simulink model "ROS_example"  (R2026a)
settings: Solver=FixedStepDiscrete  StopTime=tspan  FixedStep=dt_sim
values from neighbouring files (symbols this model uses):
  A = [0 1;-k/m -b/m]    [init_ROS_example.m]
  B = [0;1]    [init_ROS_example.m]
  dt_control = roundToSimTimestep(0.01,dt_sim)    [init_ROS_example.m]
  dt_data = roundToSimTimestep(1/30,dt_sim)    [init_ROS_example.m]
  dt_sim = 0.001    [init_ROS_example.m]
  x0 = [0;0]    [init_ROS_example.m]
  x_u = 1    [init_ROS_example.m]
undefined symbols (not defined in the file or in its folder): DiscIntNeverNeededParam, PID
libraries: ros2lib x6, slpidlib x1
settings Model: Creator=koryh  LastModifiedBy=koryh

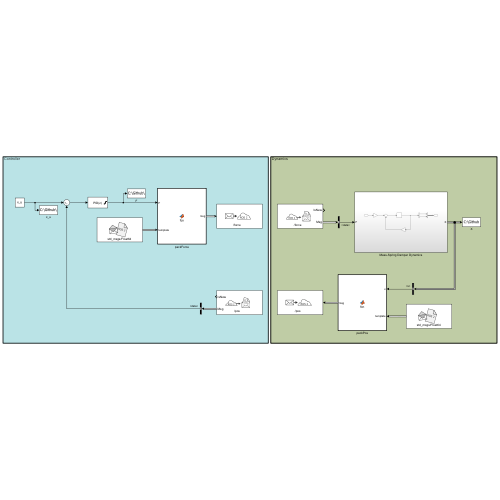
[thumbnail: Simulink's stored preview of the top-level diagram]
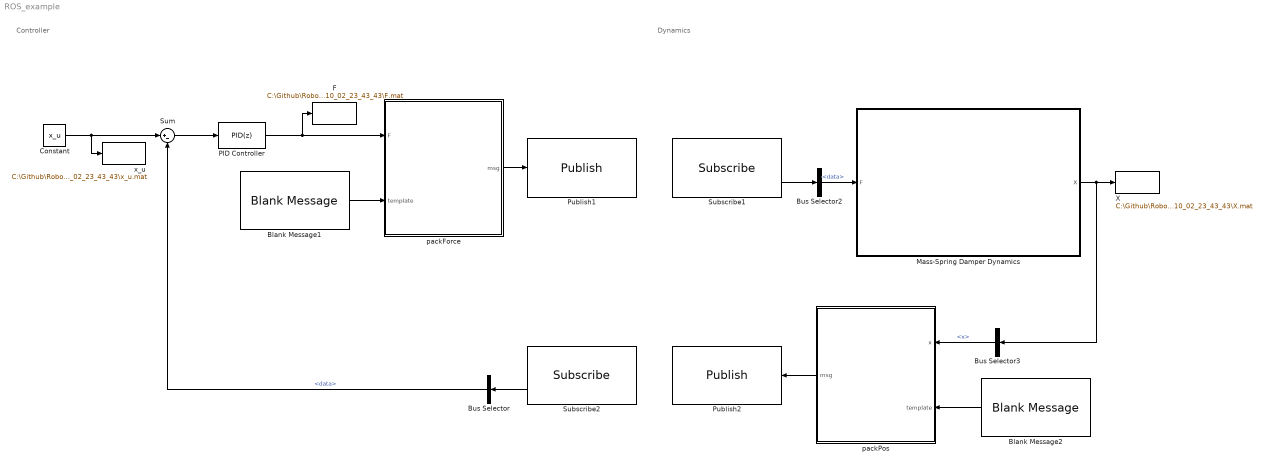
== system ROS_example ==
  note: Controller
  note: Dynamics
  Blank Message1 : ros2lib/Blank Message  messageClass=Message  entityType=std_msgs/Float64  messageType=std_msgs/Float64  SampleTime=0.01
  Blank Message2 : ros2lib/Blank Message  messageClass=Message  entityType=std_msgs/Float64  messageType=std_msgs/Float64  SampleTime=0.01
  Bus Selector : BusSelector  OutputSignals=data
  Bus Selector2 : BusSelector  OutputSignals=data
  Bus Selector3 : BusSelector  OutputSignals=x
  Constant : Constant  Value=x_u
  F : ToFile  Filename=C:\Github\Robosub\controls-onboarding-2027\examples\ROS Example\ROS_example_data\2026_10_02_23_43_43\F.mat  MatrixName=F  SaveFormat=Timeseries  SampleTime=dt_data
  Mass-Spring Damper Dynamics : Subsystem
  PID Controller : slpidlib/PID Controller  Controller=PID  Form=Parallel  TimeDomain=Discrete-time  UseExternalTs=off  SampleTime=dt_control  IntegratorMethod=Forward Euler  FilterMethod=Forward Euler  ControllerParametersSource=internal  P=PID.P  I=PID.I  UseKiTs=off  D=PID.D  UseExternalDerivativeSource=off  N=PID.N  UseFilter=on  TunerSelectOption=Transfer Function Based (PID Tuner App)  InitialConditionSource=internal  InitialConditionForIntegrator=0  InitialConditionForFilter=0  DifferentiatorICPrevScaledInput=0  ExternalReset=none  TrackingMode=off  Kt=1  LimitOutput=on  SatLimitsSource=internal  UpperSaturationLimit=PID.output_sat  LowerSaturationLimit=-PID.output_sat  LinearizeAsGain=on  AntiWindupMode=none  Kb=1  LimitIntegrator=off  UpperIntegratorSaturationLimit=inf  LowerIntegratorSaturationLimit=-inf  POutMin=[]  POutMax=[]  IOutMin=[]  IOutMax=[]  DOutMin=[]  DOutMax=[]  NOutMin=[]  NOutMax=[]  SumOutMin=[]  SumOutMax=[]  SaturationOutMin=[]  SaturationOutMax=[]  PParamMin=[]  PParamMax=[]  IParamMin=[]  IParamMax=[]  DParamMin=[]  DParamMax=[]  NParamMin=[]  NParamMax=[]  KbParamMin=[]  KbParamMax=[]  KtParamMin=[]  KtParamMax=[]  KbOutMin=[]  KbOutMax=[]  KtOutMin=[]  KtOutMax=[]  IntegratorOutMin=[]  IntegratorOutMax=[]  FilterOutMin=[]  FilterOutMax=[]  SumI1OutMin=[]  SumI1OutMax=[]  SumI2OutMin=[]  SumI2OutMax=[]  SumI3OutMin=[]  SumI3OutMax=[]  SumI4OutMin=[]  SumI4OutMax=[]  SumDOutMin=[]  SumDOutMax=[]  DifferentiatorOutMin=[]  DifferentiatorOutMax=[]  FilterDiffOutCoefMin=[]  FilterDiffOutCoefMax=[]  ReciprocalOutMin=[]  ReciprocalOutMax=[]  SumDenOutMin=[]  SumDenOutMax=[]  SumNumOutMin=[]  SumNumOutMax=[]  DivideOutMin=[]  DivideOutMax=[]  UdiffTsProdOutMin=[]  UdiffTsProdOutMax=[]  NTsProdOutMin=[]  NTsProdOutMax=[]  UintegralTsProdOutMin=[]  UintegralTsProdOutMax=[]  UngainTsProdOutMin=[]  UngainTsProdOutMax=[]  ClampingZeroOutDataTypeStr=Inherit: Inherit via back propagation  ClampingZeroOutMin=[]  ClampingZeroOutMax=[]  FilterDenConstantOutDataTypeStr=Inherit: Inherit via back propagation  FilterDenConstantOutMin=[]  FilterDenConstantOutMax=[]  PCopyOutDataTypeStr=Inherit: Inherit via back propagation  PCopyOutMin=[]  PCopyOutMax=[]  NCopyOutDataTypeStr=Inherit: Inherit via back propagation  NCopyOutMin=[]  NCopyOutMax=[]  IntegratorContinuousStateAttributes=''  IntegratorStateMustResolveToSignalObject=off  IntegratorRTWStateStorageClass=Auto  FilterContinuousStateAttributes=''  FilterStateMustResolveToSignalObject=off  FilterRTWStateStorageClass=Auto  ParallelPVariant=InternalParameters  IdealPVariant=Disabled  IVariant=InternalParameters  DVariant=InternalParameters  IntegratorVariant=Discrete  SatVariant=Enabled  AWVariant=Passthrough  PCopyVariant=Disabled  TRVariant=Disabled  FdbkBlocksVariant=Forward  IdealPFdbkVariant=Disabled  SatFdbkVariant=Disabled  DerivativeFilterVariant=ForwardEulerFilter  NVariant=InternalParameters  NCopyVariant=Disabled  FilterICVariant=InternalICsFilter  IntegratorICVariant=InternalICs  ExternalResetVariant=Disabled  TRSumVariant=Passthrough  SumFdbkVariant=Disabled  SumVariant=Sum_PID  TsampFilterVariant=InternalTs  TsampNgainVariant=Passthrough  TsampIntegralVariant=Disabled_SignalSpec  ExternalSaturationOutDataTypeStr=Inherit: Same as second input  DerivativeSourceVariant=ErrorSignal  PreIntVariant=InternalPreInt
  Publish1 : ros2lib/Publish  topicSource=Specify your own  topic=/force  messageType=std_msgs/Float64  QOSHistory=Keep last  QOSDepth=10  QOSReliability=Reliable  QOSDurability=Volatile  QOSDeadline=Inf  QOSLifespan=Inf  QOSLiveliness=Automatic  QOSLeaseDuration=Inf  QOSAvoidROSNamespaceConventions=off
  Publish2 : ros2lib/Publish  topicSource=Specify your own  topic=/pos  messageType=std_msgs/Float64  QOSHistory=Keep last  QOSDepth=10  QOSReliability=Reliable  QOSDurability=Volatile  QOSDeadline=Inf  QOSLifespan=Inf  QOSLiveliness=Automatic  QOSLeaseDuration=Inf  QOSAvoidROSNamespaceConventions=off
  Subscribe1 : ros2lib/Subscribe  topicSource=Specify your own  topic=/force  messageType=std_msgs/Float64  sampleTime=0.01  QOSHistory=Keep last  QOSDepth=10  QOSReliability=Reliable  QOSDurability=Volatile  QOSDeadline=Inf  QOSLifespan=Inf  QOSLiveliness=Automatic  QOSLeaseDuration=Inf  QOSAvoidROSNamespaceConventions=off
  Subscribe2 : ros2lib/Subscribe  topicSource=Specify your own  topic=/pos  messageType=std_msgs/Float64  sampleTime=0.01  QOSHistory=Keep last  QOSDepth=10  QOSReliability=Reliable  QOSDurability=Volatile  QOSDeadline=Inf  QOSLifespan=Inf  QOSLiveliness=Automatic  QOSLeaseDuration=Inf  QOSAvoidROSNamespaceConventions=off
  Sum : Sum  Inputs=|+-
  X : ToFile  Filename=C:\Github\Robosub\controls-onboarding-2027\examples\ROS Example\ROS_example_data\2026_10_02_23_43_43\X.mat  MatrixName=X  SaveFormat=Timeseries  SampleTime=dt_data
  packForce : MATLAB Function  TreatAsAtomicUnit=on
  packPos : MATLAB Function  TreatAsAtomicUnit=on
  x_u : ToFile  Filename=C:\Github\Robosub\controls-onboarding-2027\examples\ROS Example\ROS_example_data\2026_10_02_23_43_43\x_u.mat  MatrixName=x_u  SaveFormat=Timeseries  SampleTime=dt_data
  wires:
  Subscribe1/2 -> Bus Selector2/1
  Bus Selector2/1 -> Mass-Spring Damper Dynamics/1(F)  "<data>"
  Mass-Spring Damper Dynamics/1(X) -> X/1, Bus Selector3/1
  Sum/1 -> PID Controller/1
  Constant/1 -> x_u/1, Sum/1
  PID Controller/1 -> packForce/1(F), F/1
  packForce/1(msg) -> Publish1/1
  Blank Message1/1 -> packForce/2(template)
  packPos/1(msg) -> Publish2/1
  Bus Selector3/1 -> packPos/1(x)  "<x>"
  Blank Message2/1 -> packPos/2(template)
  Subscribe2/2 -> Bus Selector/1
  Bus Selector/1 -> Sum/2  "<data>"

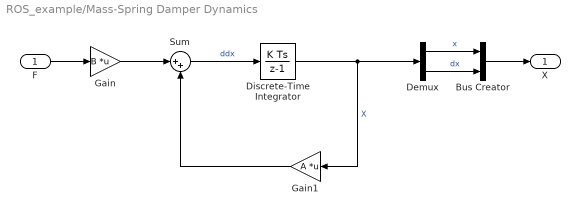
== system ROS_example/Mass-Spring Damper Dynamics ==
  F : Inport  SampleTime=dt_sim
  Bus Creator : BusCreator  Inputs=2
  Demux : Demux  Outputs=2
  Discrete-Time Integrator : DiscreteIntegrator  InitialCondition=x0  SampleTime=-1  ICPrevOutput=DiscIntNeverNeededParam  ICPrevScaledInput=DiscIntNeverNeededParam
  Gain : Gain  Gain=B  Multiplication=Matrix(K*u)
  Gain1 : Gain  Gain=A  Multiplication=Matrix(K*u)
  Sum : Sum  Inputs=|++
  X : Outport
  wires:
  F/1 -> Gain/1
  Gain/1 -> Sum/1
  Sum/1 -> Discrete-Time Integrator/1  "ddx"
  Discrete-Time Integrator/1 -> Demux/1, Gain1/1  "X"
  Gain1/1 -> Sum/2
  Demux/1 -> Bus Creator/1  "x"
  Demux/2 -> Bus Creator/2  "dx"
  Bus Creator/1 -> X/1

== matlab function ROS_example/packPos ==
  settings: updateMethod=DISCRETE  sampleTime=dt_control
  data: x input; msg output Bus: SL_Bus_std_msgs_Float64; template input Bus: SL_Bus_std_msgs_Float64
function msg = fcn(x, template)

msg = template;

msg.data = x;

== matlab function ROS_example/packForce ==
  settings: updateMethod=DISCRETE  sampleTime=dt_control
  data: F input; msg output Bus: SL_Bus_std_msgs_Float64; template input Bus: SL_Bus_std_msgs_Float64
function msg = fcn(F, template)

msg = template;

msg.data = F;
